simulink model "stm32f4_uart_hostpc_target_demo"  (Simulink 8.2)
settings: Solver=FixedStepDiscrete  SolverMode=SingleTasking  StartTime=0.0  StopTime=10.0  RelTol=1e-3
PreLoadFcn:
  | waijung.modelPreload; % Required for working with Waijung Blockset. Do not remove.
undefined symbols (not defined in the file): HSEOSC, Link, LQFP176, ST, STM32F417IG
libraries: stm32f4_io_lib x1, stm32f4_adc_lib x1, stm32f4_device_config_lib x1
CloseFcn:
  | waijung.modelClose; % Required for working with Waijung Blockset. Do not remove.
settings Model: Creator=Krisada  LastModifiedBy=Krisada
settings OptimizationCC: OptimizeModelRefInitCode=on  LifeSpan=1
settings DebuggingCC: ParameterPrecisionLossMsg=none
settings HardwareCC: ProdEndianess=LittleEndian  ProdHWDeviceType=ARM Compatible->Cortex - M4  TargetEndianess=LittleEndian  TargetHWDeviceType=ARM Compatible->Cortex - M4
settings RTWCC: SystemTargetFile=stm32f4.tlc  GenerateMakefile=off  TemplateMakefile=ert_default_tmf  Description=STM32F4 Target  ProcessScript=stm32f4_make_rtw_hook
settings CodeAppCC: IgnoreCustomStorageClasses=off  CustomSymbolStrType=$N$R$M  InternalIdentifier=Classic
settings STFCustomTargetCC: CodeReplacementLibrary=ANSI_C  ModelReferenceCompliant=off  CombineOutputUpdateFcns=on  ERTCustomFileBanners=on  SupportContinuousTime=off  SupportNonInlinedSFcns=off  MATLABClassNameForMDSCustomization=Simulink.SoftwareTarget.ERTCustomization  GRTInterface=off  SystemTargetFile=stm32f4.tlc
settings ERTTargetCC: CodeReplacementLibrary=ANSI_C  MultiwordLength=2048  ModelReferenceCompliant=off  ParMdlRefBuildCompliant=off  CompOptLevelCompliant=off  ConcurrentExecutionCompliant=off  ERTFirstTimeCompliant=off  ModelStepFunctionPrototypeControlCompliant=off  CPPClassGenCompliant=off  ExtModeMexFile=noextcomm  InlinedParameterPlacement=NonHierarchical  ERTSrcFileBannerTemplate=stm32f4_code_template.cgt  ERTHdrFileBannerTemplate=stm32f4_code_template.cgt  ERTDataSrcFileTemplate=stm32f4_code_template.cgt  ERTDataHdrFileTemplate=stm32f4_code_template.cgt  ERTCustomFileTemplate=stm32f4_file_process.tlc  ConvertIfToSwitch=off  SuppressUnreachableDefaultCases=off

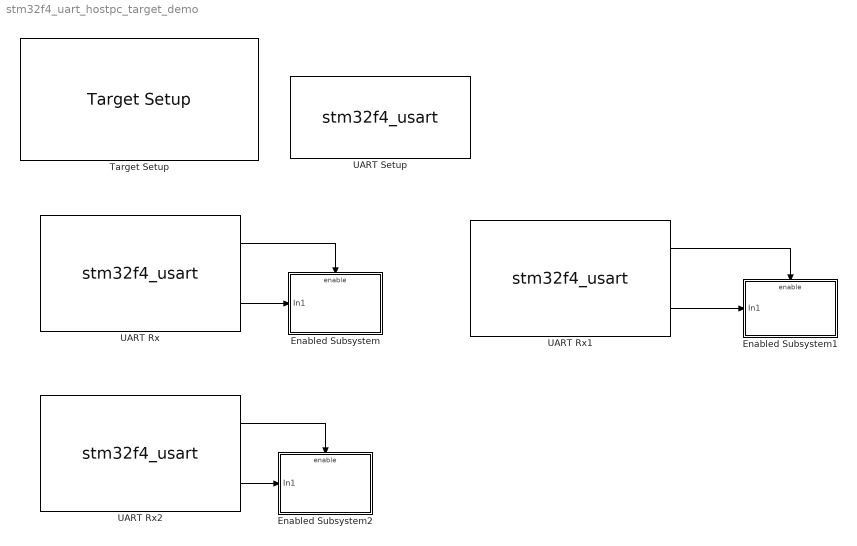
== system stm32f4_uart_hostpc_target_demo ==
  Enabled Subsystem : Subsystem  TreatAsAtomicUnit=on
  Enabled Subsystem1 : Subsystem  TreatAsAtomicUnit=on
  Enabled Subsystem2 : Subsystem  TreatAsAtomicUnit=on
  Target Setup : stm32f4_device_config_lib/Target Setup  Priority=100  compiler=GNU ARM  previous_compiler=GNU ARM  mcu=STM32F417IG (LQFP176)  mcustr=STM32F417IG  clockconfig=HSEOSC-8MHz  system_stm32f4xx_c_path=F:\trunk\targets\stm32f4_target\stm32f4\utils\system_stm32f4xx_default\STM32F40_41xxx\hseosc8mhz  showmemoryconfiguration=off  stacksize=0x400  heapsize=0x200  enableautocompiledownload=on  fullchiperase=off  programmerinterface=ST-Link  editctrlstr=on  compilercontrolstr=$(patsubst %, -I%, .) -mcpu=cortex-m4 -mthumb -mthumb-interwork -mfloat-abi=hard -mfpu=fpv4-sp-d16 -ffast-math -Wall -Wextra -Ofast  assemblercontrolstr=$(patsubst %, -I%, .) -mcpu=cortex-m4 -mthumb -mthumb-interwork -mfloat-abi=hard -mfpu=fpv4-sp-d16 -ffast-math -Wall -Wextra -Ofast -Wa,-amhls=$(<:.s=.lst) -D__STACK_SIZE=$(STACK_SIZE) -D__HEAP_SIZE=$(HEAP_SIZE)  linkercontrolstr=-T$(LD_SCRIPT) -g -Wl,-Map=$(MAP),--cref,--no-warn-mismatch -mcpu=cortex-m4 -mthumb -mthumb-interwork -mfloat-abi=hard -mfpu=fpv4-sp-d16 -specs=nosys.specs  runafterdownload=on  execprofile=None  profileruart=1  profilerbaud=115200  profilertxpin=D8  profilerinitstr=0.01,168000000,1680000,115200,0  manualsetsampletime=off  sampletime=0.01  blockid=TargetSetup  systickreloadvalue=1680000  hseval=8000000  lastprofileruart=1  hclk=168000000  flashorigin=0x8000000  flashlength=1024k  ramorigin=0x20000000  ramlength=128k  useextram=off
  UART Rx : S-Function  Priority=1  FunctionName=stm32f4_usart  Parameters=configuration,uartmodule,transfer,baudrate,inputtype,outputtype,confstr,binheaderarray,binterminatorarray,asciiheader,asciiterminator,bindatalength,packetmode,varname,sampletime,sampletimestr,blockid  EnableBusSupport=off  mask(stm32f4_usart){configuration=Rx, uartmodule=3, baudrate=115200, databits=8, parity=No, stopbit=1, remaptxpin=Not used, remaprxpin=Not used, flowcontrol=None, remapctspin=Not used, remaprtspin=Not used, advanceoptions=off, rxbuffersize=512, txbuffersize=512, transfer=Non-Blocking, packetmode=Ascii, binheader='7E 7E', binterminator='03 03', porttype_double=1, porttype_single=0, porttype_int8=1, porttype_uint8=0, porttype_int16=0, porttype_uint16=0, porttype_int32=0, porttype_uint32=0, asciiformat='LED1=%u', rx_asciiterminator=CR (0x0D - "\r"), tx_asciiterminator=LF (0x0A - "\n"), storagename=D0, varname=, inputtype=[0], outputtype=[2 3  7], binheaderarray=[0], binterminatorarray=[0], bindatalength=0, asciiheader='LED1=%u\r', asciiterminator=[1 13], sampletime=0.01, sampletimestr=0.01, blockid=UARTRx, confstr=[ "dummy", "0", "*", "*", "0", "*", "*", "0", "*", "*", "0", "*", "*", "1", "4", "3", "1", "4", "1", "512", "512", "1", "3", "115200", "8", "No", "1", "None", "USART3"], lastmodule=1}
      mask prompts: uartmodule "UART Module"; baudrate "Baud rate (bps)"; databits "Data bits"; stopbit "Stop bit"; remaptxpin "Tx Pin"; remaprxpin "Rx Pin"; flowcontrol "Hardware flow control"; remapctspin "HW Flow control, CTS Pin"; remaprtspin "HW Flow control, RTS Pin"; advanceoptions "Advance options"; rxbuffersize "Rx buffer size (bytes)"; txbuffersize "Tx buffer size (bytes)"; packetmode "Packet mode"; binheader "Binary header (example: '7E 7E')"; binterminator "Binary terminator (example: '03 03')"; porttype_double "Number of data port, type DOUBLE"; porttype_single "Number of data port, type SINGLE"; porttype_int8 "Number of data port, type INT8"; porttype_uint8 "Number of data port, type UINT8"; porttype_int16 "Number of data port, type INT16"; porttype_uint16 "Number of data port, type UINT16"; porttype_int32 "Number of data port, type INT32"; porttype_uint32 "Number of data port, type UINT32"; asciiformat "Ascii format"; rx_asciiterminator "End of packet"; tx_asciiterminator "End of packet"; storagename "Buffer"; varname "Var name"; inputtype "Input data type"; outputtype "Output data type"; binheaderarray "Binary header"; binterminatorarray "Binary terminator"; bindatalength "Binary data length"; asciiheader "Ascii header (printf format)"; asciiterminator "Ascii terminator"; sampletime "Sample time (sec)"; sampletimestr "Compiled sample time (sec) in string"; confstr "Configuration string"; lastmodule "Last module selected"
      mask init:
      | stm32f4_usart_callback('init');
      mask Help: web(fullfile(waijungdocroot,'stm32f4_usart_rx.htm'), '-browser')
      mask TypeOptions configuration: Setup | Tx | Rx
      mask Callback configuration: stm32f4_usart_callback('configuration');
      mask TypeOptions uartmodule: 1 | 2 | 3 | 4 | 5 | 6
      mask Callback uartmodule: stm32f4_usart_callback('uartmodule');
      mask Callback baudrate: stm32f4_usart_callback('baudrate');
      mask TypeOptions databits: 8
      mask TypeOptions parity: No | Odd | Even
      mask TypeOptions stopbit: 0.5 | 1 | 1.5 | 2
      mask TypeOptions remaptxpin: Not used | A9 | B6
      mask TypeOptions remaprxpin: Not used | A10 | B7
      mask TypeOptions flowcontrol: None | RTS | CTS | RTS/CTS
      mask Callback flowcontrol: stm32f4_usart_callback('flowcontrol');
      mask TypeOptions remapctspin: Not used | A11
      mask TypeOptions remaprtspin: Not used | A12
      mask Callback advanceoptions: stm32f4_usart_callback('advanceoptions');
      mask TypeOptions rxbuffersize: 16 | 32 | 64 | 128 | 256 | 512 | 1024 | 2048
      mask TypeOptions txbuffersize: 16 | 32 | 64 | 128 | 256 | 512 | 1024 | 2048
      mask TypeOptions transfer: Blocking | Non-Blocking
      mask Callback transfer: stm32f4_usart_callback('transfer');
      mask TypeOptions packetmode: Ascii | Binary | String Buffer
      mask Callback packetmode: stm32f4_usart_callback('packetmode');
      mask Callback binheader: stm32f4_usart_callback('binheader');
      mask Callback binterminator: stm32f4_usart_callback('binterminator');
      mask Callback porttype_double: stm32f4_usart_callback('porttype');
      mask Callback porttype_single: stm32f4_usart_callback('porttype');
      mask Callback porttype_int8: stm32f4_usart_callback('porttype');
      mask Callback porttype_uint8: stm32f4_usart_callback('porttype');
      mask Callback porttype_int16: stm32f4_usart_callback('porttype');
      mask Callback porttype_uint16: stm32f4_usart_callback('porttype');
      mask Callback porttype_int32: stm32f4_usart_callback('porttype');
      mask Callback porttype_uint32: stm32f4_usart_callback('porttype');
      mask Callback asciiformat: stm32f4_usart_callback('asciiformat');
      mask TypeOptions rx_asciiterminator: CR (0x0D - "\r") | LF (0x0A - "\n") | CRLF (0x0D 0x0A - "\r\n")
      mask Callback rx_asciiterminator: stm32f4_usart_callback('rx_asciiterminator');
      mask TypeOptions tx_asciiterminator: CR (0x0D - "\r") | LF (0x0A - "\n") | CRLF (0x0D 0x0A - "\r\n") | None
      mask Callback tx_asciiterminator: stm32f4_usart_callback('tx_asciiterminator');
      mask TypeOptions storagename: D0
      mask Callback storagename: stm32f4_usart_callback('storagename');
      mask Callback varname: stm32f4_usart_callback('varname');
      mask Callback sampletime: stm32f4_usart_callback('sampletime');
      mask Callback sampletimestr: stm32f4_usart_callback('sampletimestr');
      mask Callback blockid: stm32f4_usart_callback('blockid');
      mask Display: text(0.05, 0.5, 'Module: USART3_Rx\nPacket: Ascii\nTransfer: Non-Blocking\nTs (sec): 0.01','ver','middle','hor','left'); port_label('output', 1,'READY'); port_label('output', 2,'uint32');
  UART Rx1 : S-Function  Priority=1  FunctionName=stm32f4_usart  Parameters=configuration,uartmodule,transfer,baudrate,inputtype,outputtype,confstr,binheaderarray,binterminatorarray,asciiheader,asciiterminator,bindatalength,packetmode,varname,sampletime,sampletimestr,blockid  EnableBusSupport=off  mask(stm32f4_usart){configuration=Rx, uartmodule=3, baudrate=115200, databits=8, parity=No, stopbit=1, remaptxpin=Not used, remaprxpin=Not used, flowcontrol=None, remapctspin=Not used, remaprtspin=Not used, advanceoptions=off, rxbuffersize=512, txbuffersize=512, transfer=Non-Blocking, packetmode=Ascii, binheader='7E 7E', binterminator='03 03', porttype_double=1, porttype_single=0, porttype_int8=1, porttype_uint8=0, porttype_int16=0, porttype_uint16=0, porttype_int32=0, porttype_uint32=0, asciiformat='ADC%u?', rx_asciiterminator=CR (0x0D - "\r"), tx_asciiterminator=LF (0x0A - "\n"), storagename=<empty>, varname=, inputtype=[0], outputtype=[2 3  7], binheaderarray=[0], binterminatorarray=[0], bindatalength=0, asciiheader='ADC%u?\r', asciiterminator=[1 13], sampletime=0.01, sampletimestr=0.01, blockid=UARTRx1, confstr=[ "dummy", "0", "*", "*", "0", "*", "*", "0", "*", "*", "0", "*", "*", "1", "4", "3", "1", "4", "1", "512", "512", "1", "3", "115200", "8", "No", "1", "None", "USART3"], lastmodule=1}
      mask prompts: uartmodule "UART Module"; baudrate "Baud rate (bps)"; databits "Data bits"; stopbit "Stop bit"; remaptxpin "Tx Pin"; remaprxpin "Rx Pin"; flowcontrol "Hardware flow control"; remapctspin "HW Flow control, CTS Pin"; remaprtspin "HW Flow control, RTS Pin"; advanceoptions "Advance options"; rxbuffersize "Rx buffer size (bytes)"; txbuffersize "Tx buffer size (bytes)"; packetmode "Packet mode"; binheader "Binary header (example: '7E 7E')"; binterminator "Binary terminator (example: '03 03')"; porttype_double "Number of data port, type DOUBLE"; porttype_single "Number of data port, type SINGLE"; porttype_int8 "Number of data port, type INT8"; porttype_uint8 "Number of data port, type UINT8"; porttype_int16 "Number of data port, type INT16"; porttype_uint16 "Number of data port, type UINT16"; porttype_int32 "Number of data port, type INT32"; porttype_uint32 "Number of data port, type UINT32"; asciiformat "Ascii format"; rx_asciiterminator "End of packet"; tx_asciiterminator "End of packet"; storagename "Buffer"; varname "Var name"; inputtype "Input data type"; outputtype "Output data type"; binheaderarray "Binary header"; binterminatorarray "Binary terminator"; bindatalength "Binary data length"; asciiheader "Ascii header (printf format)"; asciiterminator "Ascii terminator"; sampletime "Sample time (sec)"; sampletimestr "Compiled sample time (sec) in string"; confstr "Configuration string"; lastmodule "Last module selected"
      mask init:
      | stm32f4_usart_callback('init');
      mask Help: web(fullfile(waijungdocroot,'stm32f4_usart_rx.htm'), '-browser')
      mask TypeOptions configuration: Setup | Tx | Rx
      mask Callback configuration: stm32f4_usart_callback('configuration');
      mask TypeOptions uartmodule: 1 | 2 | 3 | 4 | 5 | 6
      mask Callback uartmodule: stm32f4_usart_callback('uartmodule');
      mask Callback baudrate: stm32f4_usart_callback('baudrate');
      mask TypeOptions databits: 8
      mask TypeOptions parity: No | Odd | Even
      mask TypeOptions stopbit: 0.5 | 1 | 1.5 | 2
      mask TypeOptions remaptxpin: Not used | A9 | B6
      mask TypeOptions remaprxpin: Not used | A10 | B7
      mask TypeOptions flowcontrol: None | RTS | CTS | RTS/CTS
      mask Callback flowcontrol: stm32f4_usart_callback('flowcontrol');
      mask TypeOptions remapctspin: Not used | A11
      mask TypeOptions remaprtspin: Not used | A12
      mask Callback advanceoptions: stm32f4_usart_callback('advanceoptions');
      mask TypeOptions rxbuffersize: 16 | 32 | 64 | 128 | 256 | 512 | 1024 | 2048
      mask TypeOptions txbuffersize: 16 | 32 | 64 | 128 | 256 | 512 | 1024 | 2048
      mask TypeOptions transfer: Blocking | Non-Blocking
      mask Callback transfer: stm32f4_usart_callback('transfer');
      mask TypeOptions packetmode: Ascii | Binary | String Buffer
      mask Callback packetmode: stm32f4_usart_callback('packetmode');
      mask Callback binheader: stm32f4_usart_callback('binheader');
      mask Callback binterminator: stm32f4_usart_callback('binterminator');
      mask Callback porttype_double: stm32f4_usart_callback('porttype');
      mask Callback porttype_single: stm32f4_usart_callback('porttype');
      mask Callback porttype_int8: stm32f4_usart_callback('porttype');
      mask Callback porttype_uint8: stm32f4_usart_callback('porttype');
      mask Callback porttype_int16: stm32f4_usart_callback('porttype');
      mask Callback porttype_uint16: stm32f4_usart_callback('porttype');
      mask Callback porttype_int32: stm32f4_usart_callback('porttype');
      mask Callback porttype_uint32: stm32f4_usart_callback('porttype');
      mask Callback asciiformat: stm32f4_usart_callback('asciiformat');
      mask TypeOptions rx_asciiterminator: CR (0x0D - "\r") | LF (0x0A - "\n") | CRLF (0x0D 0x0A - "\r\n")
      mask Callback rx_asciiterminator: stm32f4_usart_callback('rx_asciiterminator');
      mask TypeOptions tx_asciiterminator: CR (0x0D - "\r") | LF (0x0A - "\n") | CRLF (0x0D 0x0A - "\r\n") | None
      mask Callback tx_asciiterminator: stm32f4_usart_callback('tx_asciiterminator');
      mask TypeOptions storagename: <empty>
      mask Callback storagename: stm32f4_usart_callback('storagename');
      mask Callback varname: stm32f4_usart_callback('varname');
      mask Callback sampletime: stm32f4_usart_callback('sampletime');
      mask Callback sampletimestr: stm32f4_usart_callback('sampletimestr');
      mask Callback blockid: stm32f4_usart_callback('blockid');
      mask Display: text(0.05, 0.5, 'Module: USART3_Rx\nPacket: Ascii\nTransfer: Non-Blocking\nTs (sec): 0.01','ver','middle','hor','left'); port_label('output', 1,'READY'); port_label('output', 2,'uint32');
  UART Rx2 : S-Function  Priority=1  FunctionName=stm32f4_usart  Parameters=configuration,uartmodule,transfer,baudrate,inputtype,outputtype,confstr,binheaderarray,binterminatorarray,asciiheader,asciiterminator,bindatalength,packetmode,varname,sampletime,sampletimestr,blockid  EnableBusSupport=off  mask(stm32f4_usart){configuration=Rx, uartmodule=3, baudrate=115200, databits=8, parity=No, stopbit=1, remaptxpin=Not used, remaprxpin=Not used, flowcontrol=None, remapctspin=Not used, remaprtspin=Not used, advanceoptions=off, rxbuffersize=512, txbuffersize=512, transfer=Non-Blocking, packetmode=Ascii, binheader='7E 7E', binterminator='03 03', porttype_double=1, porttype_single=0, porttype_int8=1, porttype_uint8=0, porttype_int16=0, porttype_uint16=0, porttype_int32=0, porttype_uint32=0, asciiformat='Input %f', rx_asciiterminator=CR (0x0D - "\r"), tx_asciiterminator=LF (0x0A - "\n"), storagename=<empty>, varname=, inputtype=[0], outputtype=[2 3  1], binheaderarray=[0], binterminatorarray=[0], bindatalength=0, asciiheader='Input %f\r', asciiterminator=[1 13], sampletime=0.01, sampletimestr=0.01, blockid=UARTRx2, confstr=[ "dummy", "0", "*", "*", "0", "*", "*", "0", "*", "*", "0", "*", "*", "1", "4", "3", "1", "4", "1", "512", "512", "1", "3", "115200", "8", "No", "1", "None", "USART3"], lastmodule=1}
      mask prompts: uartmodule "UART Module"; baudrate "Baud rate (bps)"; databits "Data bits"; stopbit "Stop bit"; remaptxpin "Tx Pin"; remaprxpin "Rx Pin"; flowcontrol "Hardware flow control"; remapctspin "HW Flow control, CTS Pin"; remaprtspin "HW Flow control, RTS Pin"; advanceoptions "Advance options"; rxbuffersize "Rx buffer size (bytes)"; txbuffersize "Tx buffer size (bytes)"; packetmode "Packet mode"; binheader "Binary header (example: '7E 7E')"; binterminator "Binary terminator (example: '03 03')"; porttype_double "Number of data port, type DOUBLE"; porttype_single "Number of data port, type SINGLE"; porttype_int8 "Number of data port, type INT8"; porttype_uint8 "Number of data port, type UINT8"; porttype_int16 "Number of data port, type INT16"; porttype_uint16 "Number of data port, type UINT16"; porttype_int32 "Number of data port, type INT32"; porttype_uint32 "Number of data port, type UINT32"; asciiformat "Ascii format"; rx_asciiterminator "End of packet"; tx_asciiterminator "End of packet"; storagename "Buffer"; varname "Var name"; inputtype "Input data type"; outputtype "Output data type"; binheaderarray "Binary header"; binterminatorarray "Binary terminator"; bindatalength "Binary data length"; asciiheader "Ascii header (printf format)"; asciiterminator "Ascii terminator"; sampletime "Sample time (sec)"; sampletimestr "Compiled sample time (sec) in string"; confstr "Configuration string"; lastmodule "Last module selected"
      mask init:
      | stm32f4_usart_callback('init');
      mask Help: web(fullfile(waijungdocroot,'stm32f4_usart_rx.htm'), '-browser')
      mask TypeOptions configuration: Setup | Tx | Rx
      mask Callback configuration: stm32f4_usart_callback('configuration');
      mask TypeOptions uartmodule: 1 | 2 | 3 | 4 | 5 | 6
      mask Callback uartmodule: stm32f4_usart_callback('uartmodule');
      mask Callback baudrate: stm32f4_usart_callback('baudrate');
      mask TypeOptions databits: 8
      mask TypeOptions parity: No | Odd | Even
      mask TypeOptions stopbit: 0.5 | 1 | 1.5 | 2
      mask TypeOptions remaptxpin: Not used | A9 | B6
      mask TypeOptions remaprxpin: Not used | A10 | B7
      mask TypeOptions flowcontrol: None | RTS | CTS | RTS/CTS
      mask Callback flowcontrol: stm32f4_usart_callback('flowcontrol');
      mask TypeOptions remapctspin: Not used | A11
      mask TypeOptions remaprtspin: Not used | A12
      mask Callback advanceoptions: stm32f4_usart_callback('advanceoptions');
      mask TypeOptions rxbuffersize: 16 | 32 | 64 | 128 | 256 | 512 | 1024 | 2048
      mask TypeOptions txbuffersize: 16 | 32 | 64 | 128 | 256 | 512 | 1024 | 2048
      mask TypeOptions transfer: Blocking | Non-Blocking
      mask Callback transfer: stm32f4_usart_callback('transfer');
      mask TypeOptions packetmode: Ascii | Binary | String Buffer
      mask Callback packetmode: stm32f4_usart_callback('packetmode');
      mask Callback binheader: stm32f4_usart_callback('binheader');
      mask Callback binterminator: stm32f4_usart_callback('binterminator');
      mask Callback porttype_double: stm32f4_usart_callback('porttype');
      mask Callback porttype_single: stm32f4_usart_callback('porttype');
      mask Callback porttype_int8: stm32f4_usart_callback('porttype');
      mask Callback porttype_uint8: stm32f4_usart_callback('porttype');
      mask Callback porttype_int16: stm32f4_usart_callback('porttype');
      mask Callback porttype_uint16: stm32f4_usart_callback('porttype');
      mask Callback porttype_int32: stm32f4_usart_callback('porttype');
      mask Callback porttype_uint32: stm32f4_usart_callback('porttype');
      mask Callback asciiformat: stm32f4_usart_callback('asciiformat');
      mask TypeOptions rx_asciiterminator: CR (0x0D - "\r") | LF (0x0A - "\n") | CRLF (0x0D 0x0A - "\r\n")
      mask Callback rx_asciiterminator: stm32f4_usart_callback('rx_asciiterminator');
      mask TypeOptions tx_asciiterminator: CR (0x0D - "\r") | LF (0x0A - "\n") | CRLF (0x0D 0x0A - "\r\n") | None
      mask Callback tx_asciiterminator: stm32f4_usart_callback('tx_asciiterminator');
      mask TypeOptions storagename: <empty>
      mask Callback storagename: stm32f4_usart_callback('storagename');
      mask Callback varname: stm32f4_usart_callback('varname');
      mask Callback sampletime: stm32f4_usart_callback('sampletime');
      mask Callback sampletimestr: stm32f4_usart_callback('sampletimestr');
      mask Callback blockid: stm32f4_usart_callback('blockid');
      mask Display: text(0.05, 0.5, 'Module: USART3_Rx\nPacket: Ascii\nTransfer: Non-Blocking\nTs (sec): 0.01','ver','middle','hor','left'); port_label('output', 1,'READY'); port_label('output', 2,'single');
  UART Setup : S-Function  Priority=1  FunctionName=stm32f4_usart  Parameters=configuration,uartmodule,transfer,baudrate,inputtype,outputtype,confstr,binheaderarray,binterminatorarray,asciiheader,asciiterminator,bindatalength,packetmode,varname,sampletime,sampletimestr,blockid  EnableBusSupport=off  mask(stm32f4_usart){configuration=Setup, uartmodule=3, baudrate=115200, databits=8, parity=No, stopbit=1, remaptxpin=D8, remaprxpin=D9, flowcontrol=None, remapctspin=Not used, remaprtspin=Not used, advanceoptions=off, rxbuffersize=512, txbuffersize=512, transfer=Blocking, packetmode=Ascii, binheader='7E 7E', binterminator='03 03', porttype_double=1, porttype_single=0, porttype_int8=1, porttype_uint8=0, porttype_int16=0, porttype_uint16=0, porttype_int32=0, porttype_uint32=0, asciiformat='%d,%f', rx_asciiterminator=CRLF (0x0D 0x0A - "\r\n"), tx_asciiterminator=CR (0x0D - "\r"), storagename=<empty>, varname=, inputtype=[0], outputtype=[0], binheaderarray=[0], binterminatorarray=[0], bindatalength=0, asciiheader='', asciiterminator=[0], sampletime=-1, sampletimestr=0.01, blockid=UARTSetup, confstr=[ "dummy", "1", "D", "8", "1", "D", "9", "0", "*", "*", "0", "*", "*", "1", "4", "3", "1", "4", "1", "512", "512", "1", "3", "115200", "8", "No", "1", "None", "USART3"], lastmodule=3}
      mask prompts: uartmodule "UART Module"; baudrate "Baud rate (bps)"; databits "Data bits"; stopbit "Stop bit"; remaptxpin "Tx Pin"; remaprxpin "Rx Pin"; flowcontrol "Hardware flow control"; remapctspin "HW Flow control, CTS Pin"; remaprtspin "HW Flow control, RTS Pin"; advanceoptions "Advance options"; rxbuffersize "Rx buffer size (bytes)"; txbuffersize "Tx buffer size (bytes)"; packetmode "Packet mode"; binheader "Binary header (example: '7E 7E')"; binterminator "Binary terminator (example: '03 03')"; porttype_double "Number of data port, type DOUBLE"; porttype_single "Number of data port, type SINGLE"; porttype_int8 "Number of data port, type INT8"; porttype_uint8 "Number of data port, type UINT8"; porttype_int16 "Number of data port, type INT16"; porttype_uint16 "Number of data port, type UINT16"; porttype_int32 "Number of data port, type INT32"; porttype_uint32 "Number of data port, type UINT32"; asciiformat "Ascii format"; rx_asciiterminator "End of packet"; tx_asciiterminator "End of packet"; storagename "Buffer"; varname "Var name"; inputtype "Input data type"; outputtype "Output data type"; binheaderarray "Binary header"; binterminatorarray "Binary terminator"; bindatalength "Binary data length"; asciiheader "Ascii header (printf format)"; asciiterminator "Ascii terminator"; sampletime "Sample time (sec)"; sampletimestr "Compiled sample time (sec) in string"; confstr "Configuration string"; lastmodule "Last module selected"
      mask init:
      | stm32f4_usart_callback('init');
      mask Help: web(fullfile(waijungdocroot,'stm32f4_usart_setup.htm'), '-browser')
      mask TypeOptions configuration: Setup | Tx | Rx
      mask Callback configuration: stm32f4_usart_callback('configuration');
      mask TypeOptions uartmodule: 1 | 2 | 3 | 4 | 5 | 6
      mask Callback uartmodule: stm32f4_usart_callback('uartmodule');
      mask Callback baudrate: stm32f4_usart_callback('baudrate');
      mask TypeOptions databits: 8
      mask TypeOptions parity: No | Odd | Even
      mask TypeOptions stopbit: 0.5 | 1 | 1.5 | 2
      mask TypeOptions remaptxpin: Not used | B10 | C10 | D8
      mask TypeOptions remaprxpin: Not used | B11 | C11 | D9
      mask TypeOptions flowcontrol: None | RTS | CTS | RTS/CTS
      mask Callback flowcontrol: stm32f4_usart_callback('flowcontrol');
      mask TypeOptions remapctspin: Not used | B13 | D11
      mask TypeOptions remaprtspin: Not used | B14 | D12
      mask Callback advanceoptions: stm32f4_usart_callback('advanceoptions');
      mask TypeOptions rxbuffersize: 16 | 32 | 64 | 128 | 256 | 512 | 1024 | 2048
      mask TypeOptions txbuffersize: 16 | 32 | 64 | 128 | 256 | 512 | 1024 | 2048
      mask TypeOptions transfer: Blocking | Non-Blocking
      mask Callback transfer: stm32f4_usart_callback('transfer');
      mask TypeOptions packetmode: Ascii | Binary | String Buffer
      mask Callback packetmode: stm32f4_usart_callback('packetmode');
      mask Callback binheader: stm32f4_usart_callback('binheader');
      mask Callback binterminator: stm32f4_usart_callback('binterminator');
      mask Callback porttype_double: stm32f4_usart_callback('porttype');
      mask Callback porttype_single: stm32f4_usart_callback('porttype');
      mask Callback porttype_int8: stm32f4_usart_callback('porttype');
      mask Callback porttype_uint8: stm32f4_usart_callback('porttype');
      mask Callback porttype_int16: stm32f4_usart_callback('porttype');
      mask Callback porttype_uint16: stm32f4_usart_callback('porttype');
      mask Callback porttype_int32: stm32f4_usart_callback('porttype');
      mask Callback porttype_uint32: stm32f4_usart_callback('porttype');
      mask Callback asciiformat: stm32f4_usart_callback('asciiformat');
      mask TypeOptions rx_asciiterminator: CR (0x0D - "\r") | LF (0x0A - "\n") | CRLF (0x0D 0x0A - "\r\n")
      mask Callback rx_asciiterminator: stm32f4_usart_callback('rx_asciiterminator');
      mask TypeOptions tx_asciiterminator: CR (0x0D - "\r") | LF (0x0A - "\n") | CRLF (0x0D 0x0A - "\r\n") | None
      mask Callback tx_asciiterminator: stm32f4_usart_callback('tx_asciiterminator');
      mask TypeOptions storagename: <empty>
      mask Callback storagename: stm32f4_usart_callback('storagename');
      mask Callback varname: stm32f4_usart_callback('varname');
      mask Callback sampletime: stm32f4_usart_callback('sampletime');
      mask Callback sampletimestr: stm32f4_usart_callback('sampletimestr');
      mask Callback blockid: stm32f4_usart_callback('blockid');
      mask Display: text(0.5, 0.5, 'Module: USART3_Setup\nBaud (Bps): 115200\nDMA Buffer: 512/512\nTx/Rx Pin: D8/D9','ver','middle','hor','center');
  wires:
  UART Rx1/1 -> Enabled Subsystem1/Enable
  UART Rx1/2 -> Enabled Subsystem1/1(In1)
  UART Rx2/2 -> Enabled Subsystem2/1(In1)
  UART Rx2/1 -> Enabled Subsystem2/Enable
  UART Rx/1 -> Enabled Subsystem/Enable
  UART Rx/2 -> Enabled Subsystem/1(In1)

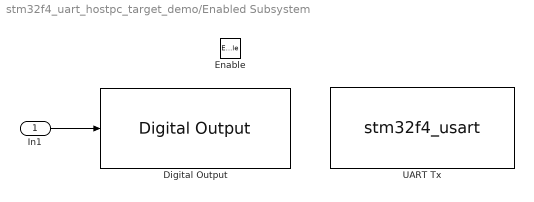
== system stm32f4_uart_hostpc_target_demo/Enabled Subsystem ==
  In1 : Inport
  Enable : EnablePort  PropagateVarSize=During execution
  Digital Output : stm32f4_io_lib/Digital Output  use_bitband=on  port=D  speed=100  porttype=Push Pull  porttypestr=PP  use_pin0=off  use_pin1=off  use_pin2=off  use_pin3=off  use_pin4=off  use_pin5=off  use_pin6=off  use_pin7=off  use_pin8=off  use_pin9=off  use_pin10=off  use_pin11=off  use_pin12=on  use_pin13=off  use_pin14=off  use_pin15=off  pinstr=GPIO_Pin_12  usedpinarray="[0  0  0  0  0  0  0  0  0  0  0  0  1  0  0  0]"  bitbandingstr="#define EnabledSubsystemDigitalOutput_D12 Peripheral_BB(GPIOD->ODR, 12)  /* Output pin */"  sampletime=-1  sampletimestr=0.01  blockid=EnabledSubsystemDigitalOutput  enablecustomportlabel=off  globalinit=off  cinputportlabel=In1, In2  coutputportlabel=0
  UART Tx : S-Function  Priority=1  FunctionName=stm32f4_usart  Parameters=configuration,uartmodule,transfer,baudrate,inputtype,outputtype,confstr,binheaderarray,binterminatorarray,asciiheader,asciiterminator,bindatalength,packetmode,varname,sampletime,sampletimestr,blockid  EnableBusSupport=off  mask(stm32f4_usart){configuration=Tx, uartmodule=3, baudrate=115200, databits=8, parity=No, stopbit=1, remaptxpin=Not used, remaprxpin=Not used, flowcontrol=None, remapctspin=Not used, remaprtspin=Not used, advanceoptions=off, rxbuffersize=512, txbuffersize=512, transfer=Blocking, packetmode=Ascii, binheader='7E 7E', binterminator='03 03', porttype_double=1, porttype_single=0, porttype_int8=1, porttype_uint8=0, porttype_int16=0, porttype_uint16=0, porttype_int32=0, porttype_uint32=0, asciiformat='Ok', rx_asciiterminator=CRLF (0x0D 0x0A - "\r\n"), tx_asciiterminator=CRLF (0x0D 0x0A - "\r\n"), storagename=<empty>, varname=, inputtype=[0 ], outputtype=[0], binheaderarray=[0], binterminatorarray=[0], bindatalength=0, asciiheader='Ok\r\n', asciiterminator=[2 13 10], sampletime=-1, sampletimestr=0.01, blockid=EnabledSubsystemUARTTx, confstr=[ "dummy", "0", "*", "*", "0", "*", "*", "0", "*", "*", "0", "*", "*", "1", "4", "3", "1", "4", "1", "512", "512", "1", "3", "115200", "8", "No", "1", "None", "USART3"], lastmodule=1}
      mask prompts: uartmodule "UART Module"; baudrate "Baud rate (bps)"; databits "Data bits"; stopbit "Stop bit"; remaptxpin "Tx Pin"; remaprxpin "Rx Pin"; flowcontrol "Hardware flow control"; remapctspin "HW Flow control, CTS Pin"; remaprtspin "HW Flow control, RTS Pin"; advanceoptions "Advance options"; rxbuffersize "Rx buffer size (bytes)"; txbuffersize "Tx buffer size (bytes)"; packetmode "Packet mode"; binheader "Binary header (example: '7E 7E')"; binterminator "Binary terminator (example: '03 03')"; porttype_double "Number of data port, type DOUBLE"; porttype_single "Number of data port, type SINGLE"; porttype_int8 "Number of data port, type INT8"; porttype_uint8 "Number of data port, type UINT8"; porttype_int16 "Number of data port, type INT16"; porttype_uint16 "Number of data port, type UINT16"; porttype_int32 "Number of data port, type INT32"; porttype_uint32 "Number of data port, type UINT32"; asciiformat "Ascii format"; rx_asciiterminator "End of packet"; tx_asciiterminator "End of packet"; storagename "Buffer"; varname "Var name"; inputtype "Input data type"; outputtype "Output data type"; binheaderarray "Binary header"; binterminatorarray "Binary terminator"; bindatalength "Binary data length"; asciiheader "Ascii header (printf format)"; asciiterminator "Ascii terminator"; sampletime "Sample time (sec)"; sampletimestr "Compiled sample time (sec) in string"; confstr "Configuration string"; lastmodule "Last module selected"
      mask init:
      | stm32f4_usart_callback('init');
      mask Help: web(fullfile(waijungdocroot,'stm32f4_usart_tx.htm'), '-browser')
      mask TypeOptions configuration: Setup | Tx | Rx
      mask Callback configuration: stm32f4_usart_callback('configuration');
      mask TypeOptions uartmodule: 1 | 2 | 3 | 4 | 5 | 6
      mask Callback uartmodule: stm32f4_usart_callback('uartmodule');
      mask Callback baudrate: stm32f4_usart_callback('baudrate');
      mask TypeOptions databits: 8
      mask TypeOptions parity: No | Odd | Even
      mask TypeOptions stopbit: 0.5 | 1 | 1.5 | 2
      mask TypeOptions remaptxpin: Not used | A9 | B6
      mask TypeOptions remaprxpin: Not used | A10 | B7
      mask TypeOptions flowcontrol: None | RTS | CTS | RTS/CTS
      mask Callback flowcontrol: stm32f4_usart_callback('flowcontrol');
      mask TypeOptions remapctspin: Not used | A11
      mask TypeOptions remaprtspin: Not used | A12
      mask Callback advanceoptions: stm32f4_usart_callback('advanceoptions');
      mask TypeOptions rxbuffersize: 16 | 32 | 64 | 128 | 256 | 512 | 1024 | 2048
      mask TypeOptions txbuffersize: 16 | 32 | 64 | 128 | 256 | 512 | 1024 | 2048
      mask TypeOptions transfer: Blocking | Non-Blocking
      mask Callback transfer: stm32f4_usart_callback('transfer');
      mask TypeOptions packetmode: Ascii | Binary | String Buffer
      mask Callback packetmode: stm32f4_usart_callback('packetmode');
      mask Callback binheader: stm32f4_usart_callback('binheader');
      mask Callback binterminator: stm32f4_usart_callback('binterminator');
      mask Callback porttype_double: stm32f4_usart_callback('porttype');
      mask Callback porttype_single: stm32f4_usart_callback('porttype');
      mask Callback porttype_int8: stm32f4_usart_callback('porttype');
      mask Callback porttype_uint8: stm32f4_usart_callback('porttype');
      mask Callback porttype_int16: stm32f4_usart_callback('porttype');
      mask Callback porttype_uint16: stm32f4_usart_callback('porttype');
      mask Callback porttype_int32: stm32f4_usart_callback('porttype');
      mask Callback porttype_uint32: stm32f4_usart_callback('porttype');
      mask Callback asciiformat: stm32f4_usart_callback('asciiformat');
      mask TypeOptions rx_asciiterminator: CR (0x0D - "\r") | LF (0x0A - "\n") | CRLF (0x0D 0x0A - "\r\n")
      mask Callback rx_asciiterminator: stm32f4_usart_callback('rx_asciiterminator');
      mask TypeOptions tx_asciiterminator: CR (0x0D - "\r") | LF (0x0A - "\n") | CRLF (0x0D 0x0A - "\r\n") | None
      mask Callback tx_asciiterminator: stm32f4_usart_callback('tx_asciiterminator');
      mask TypeOptions storagename: <empty>
      mask Callback storagename: stm32f4_usart_callback('storagename');
      mask Callback varname: stm32f4_usart_callback('varname');
      mask Callback sampletime: stm32f4_usart_callback('sampletime');
      mask Callback sampletimestr: stm32f4_usart_callback('sampletimestr');
      mask Callback blockid: stm32f4_usart_callback('blockid');
      mask Display: text(0.95, 0.5, 'Module: USART3_Tx\nPacket: Ascii\nTransfer: Blocking\nTs (sec): 0.01','ver','middle','hor','right');
  wires:
  In1/1 -> Digital Output/1

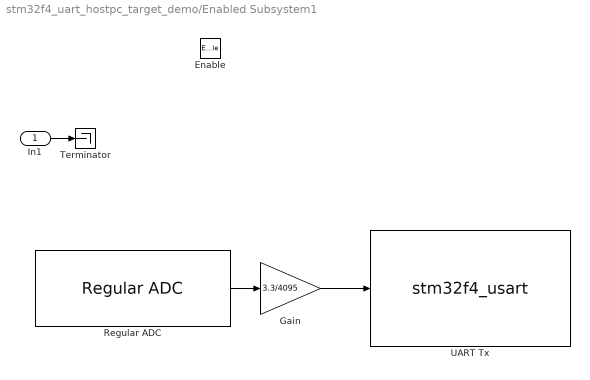
== system stm32f4_uart_hostpc_target_demo/Enabled Subsystem1 ==
  In1 : Inport
  Enable : EnablePort  PropagateVarSize=During execution
  Gain : Gain  Gain=3.3/4095  ParamDataTypeStr=single  OutDataTypeStr=single
  Regular ADC : stm32f4_adc_lib/Regular ADC  adcmodule=1  outputdatatype=Single  prescaler=2  prescalerstr=ADC_Prescaler_Div2  chsamplingtime=Auto  chsamplingtimestr=ADC_SampleTime_480Cycles  read_an0=on  read_an1=off  read_an2=off  read_an3=off  read_an4=off  read_an5=off  read_an6=off  read_an7=off  read_an8=off  read_an9=off  read_an10=off  read_an11=off  read_an12=off  read_an13=off  read_an14=off  read_an15=off  read_an16=off  read_an17=off  read_an18=off  pinstr=GPIO_Pin_0  usedpinarray="[1  0  0  0  0  0  0  0  0  0  0  0  0  0  0  0  0  0  0]"  usedportidarray=[0]  usedpinidarray=[0]  usedpinidcount=1  sampletime=0.01  blockid=EnabledSubsystem1RegularADC  enablecustomportlabel=off  cinputportlabel=0  coutputportlabel=Out1, Out2
  Terminator : Terminator
  UART Tx : S-Function  Priority=1  FunctionName=stm32f4_usart  Parameters=configuration,uartmodule,transfer,baudrate,inputtype,outputtype,confstr,binheaderarray,binterminatorarray,asciiheader,asciiterminator,bindatalength,packetmode,varname,sampletime,sampletimestr,blockid  EnableBusSupport=off  mask(stm32f4_usart){configuration=Tx, uartmodule=3, baudrate=115200, databits=8, parity=No, stopbit=1, remaptxpin=Not used, remaprxpin=Not used, flowcontrol=None, remapctspin=Not used, remaprtspin=Not used, advanceoptions=off, rxbuffersize=512, txbuffersize=512, transfer=Blocking, packetmode=Ascii, binheader='7E 7E', binterminator='03 03', porttype_double=1, porttype_single=0, porttype_int8=1, porttype_uint8=0, porttype_int16=0, porttype_uint16=0, porttype_int32=0, porttype_uint32=0, asciiformat='Reading=%f', rx_asciiterminator=CRLF (0x0D 0x0A - "\r\n"), tx_asciiterminator=CRLF (0x0D 0x0A - "\r\n"), storagename=<empty>, varname=, inputtype=[1  1], outputtype=[0], binheaderarray=[0], binterminatorarray=[0], bindatalength=0, asciiheader='Reading=%f\r\n', asciiterminator=[2 13 10], sampletime=-1, sampletimestr=0.01, blockid=EnabledSubsystem1UARTTx, confstr=[ "dummy", "0", "*", "*", "0", "*", "*", "0", "*", "*", "0", "*", "*", "1", "4", "3", "1", "4", "1", "512", "512", "1", "3", "115200", "8", "No", "1", "None", "USART3"], lastmodule=1}
      mask prompts: uartmodule "UART Module"; baudrate "Baud rate (bps)"; databits "Data bits"; stopbit "Stop bit"; remaptxpin "Tx Pin"; remaprxpin "Rx Pin"; flowcontrol "Hardware flow control"; remapctspin "HW Flow control, CTS Pin"; remaprtspin "HW Flow control, RTS Pin"; advanceoptions "Advance options"; rxbuffersize "Rx buffer size (bytes)"; txbuffersize "Tx buffer size (bytes)"; packetmode "Packet mode"; binheader "Binary header (example: '7E 7E')"; binterminator "Binary terminator (example: '03 03')"; porttype_double "Number of data port, type DOUBLE"; porttype_single "Number of data port, type SINGLE"; porttype_int8 "Number of data port, type INT8"; porttype_uint8 "Number of data port, type UINT8"; porttype_int16 "Number of data port, type INT16"; porttype_uint16 "Number of data port, type UINT16"; porttype_int32 "Number of data port, type INT32"; porttype_uint32 "Number of data port, type UINT32"; asciiformat "Ascii format"; rx_asciiterminator "End of packet"; tx_asciiterminator "End of packet"; storagename "Buffer"; varname "Var name"; inputtype "Input data type"; outputtype "Output data type"; binheaderarray "Binary header"; binterminatorarray "Binary terminator"; bindatalength "Binary data length"; asciiheader "Ascii header (printf format)"; asciiterminator "Ascii terminator"; sampletime "Sample time (sec)"; sampletimestr "Compiled sample time (sec) in string"; confstr "Configuration string"; lastmodule "Last module selected"
      mask init:
      | stm32f4_usart_callback('init');
      mask Help: web(fullfile(waijungdocroot,'stm32f4_usart_tx.htm'), '-browser')
      mask TypeOptions configuration: Setup | Tx | Rx
      mask Callback configuration: stm32f4_usart_callback('configuration');
      mask TypeOptions uartmodule: 1 | 2 | 3 | 4 | 5 | 6
      mask Callback uartmodule: stm32f4_usart_callback('uartmodule');
      mask Callback baudrate: stm32f4_usart_callback('baudrate');
      mask TypeOptions databits: 8
      mask TypeOptions parity: No | Odd | Even
      mask TypeOptions stopbit: 0.5 | 1 | 1.5 | 2
      mask TypeOptions remaptxpin: Not used | A9 | B6
      mask TypeOptions remaprxpin: Not used | A10 | B7
      mask TypeOptions flowcontrol: None | RTS | CTS | RTS/CTS
      mask Callback flowcontrol: stm32f4_usart_callback('flowcontrol');
      mask TypeOptions remapctspin: Not used | A11
      mask TypeOptions remaprtspin: Not used | A12
      mask Callback advanceoptions: stm32f4_usart_callback('advanceoptions');
      mask TypeOptions rxbuffersize: 16 | 32 | 64 | 128 | 256 | 512 | 1024 | 2048
      mask TypeOptions txbuffersize: 16 | 32 | 64 | 128 | 256 | 512 | 1024 | 2048
      mask TypeOptions transfer: Blocking | Non-Blocking
      mask Callback transfer: stm32f4_usart_callback('transfer');
      mask TypeOptions packetmode: Ascii | Binary | String Buffer
      mask Callback packetmode: stm32f4_usart_callback('packetmode');
      mask Callback binheader: stm32f4_usart_callback('binheader');
      mask Callback binterminator: stm32f4_usart_callback('binterminator');
      mask Callback porttype_double: stm32f4_usart_callback('porttype');
      mask Callback porttype_single: stm32f4_usart_callback('porttype');
      mask Callback porttype_int8: stm32f4_usart_callback('porttype');
      mask Callback porttype_uint8: stm32f4_usart_callback('porttype');
      mask Callback porttype_int16: stm32f4_usart_callback('porttype');
      mask Callback porttype_uint16: stm32f4_usart_callback('porttype');
      mask Callback porttype_int32: stm32f4_usart_callback('porttype');
      mask Callback porttype_uint32: stm32f4_usart_callback('porttype');
      mask Callback asciiformat: stm32f4_usart_callback('asciiformat');
      mask TypeOptions rx_asciiterminator: CR (0x0D - "\r") | LF (0x0A - "\n") | CRLF (0x0D 0x0A - "\r\n")
      mask Callback rx_asciiterminator: stm32f4_usart_callback('rx_asciiterminator');
      mask TypeOptions tx_asciiterminator: CR (0x0D - "\r") | LF (0x0A - "\n") | CRLF (0x0D 0x0A - "\r\n") | None
      mask Callback tx_asciiterminator: stm32f4_usart_callback('tx_asciiterminator');
      mask TypeOptions storagename: <empty>
      mask Callback storagename: stm32f4_usart_callback('storagename');
      mask Callback varname: stm32f4_usart_callback('varname');
      mask Callback sampletime: stm32f4_usart_callback('sampletime');
      mask Callback sampletimestr: stm32f4_usart_callback('sampletimestr');
      mask Callback blockid: stm32f4_usart_callback('blockid');
      mask Display: text(0.95, 0.5, 'Module: USART3_Tx\nPacket: Ascii\nTransfer: Blocking\nTs (sec): 0.01','ver','middle','hor','right'); port_label('input', 1,'single');
  wires:
  In1/1 -> Terminator/1
  Gain/1 -> UART Tx/1
  Regular ADC/1 -> Gain/1

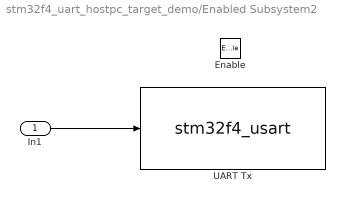
== system stm32f4_uart_hostpc_target_demo/Enabled Subsystem2 ==
  In1 : Inport
  Enable : EnablePort  PropagateVarSize=During execution
  UART Tx : S-Function  Priority=1  FunctionName=stm32f4_usart  Parameters=configuration,uartmodule,transfer,baudrate,inputtype,outputtype,confstr,binheaderarray,binterminatorarray,asciiheader,asciiterminator,bindatalength,packetmode,varname,sampletime,sampletimestr,blockid  EnableBusSupport=off  mask(stm32f4_usart){configuration=Tx, uartmodule=3, baudrate=115200, databits=8, parity=No, stopbit=1, remaptxpin=Not used, remaprxpin=Not used, flowcontrol=None, remapctspin=Not used, remaprtspin=Not used, advanceoptions=off, rxbuffersize=512, txbuffersize=512, transfer=Blocking, packetmode=Ascii, binheader='7E 7E', binterminator='03 03', porttype_double=1, porttype_single=0, porttype_int8=1, porttype_uint8=0, porttype_int16=0, porttype_uint16=0, porttype_int32=0, porttype_uint32=0, asciiformat='>>Your input is: %f', rx_asciiterminator=CRLF (0x0D 0x0A - "\r\n"), tx_asciiterminator=CRLF (0x0D 0x0A - "\r\n"), storagename=<empty>, varname=, inputtype=[1  1], outputtype=[0], binheaderarray=[0], binterminatorarray=[0], bindatalength=0, asciiheader='>>Your input is: %f\r\n', asciiterminator=[2 13 10], sampletime=-1, sampletimestr=0.01, blockid=EnabledSubsystem2UARTTx, confstr=[ "dummy", "0", "*", "*", "0", "*", "*", "0", "*", "*", "0", "*", "*", "1", "4", "3", "1", "4", "1", "512", "512", "1", "3", "115200", "8", "No", "1", "None", "USART3"], lastmodule=1}
      mask prompts: uartmodule "UART Module"; baudrate "Baud rate (bps)"; databits "Data bits"; stopbit "Stop bit"; remaptxpin "Tx Pin"; remaprxpin "Rx Pin"; flowcontrol "Hardware flow control"; remapctspin "HW Flow control, CTS Pin"; remaprtspin "HW Flow control, RTS Pin"; advanceoptions "Advance options"; rxbuffersize "Rx buffer size (bytes)"; txbuffersize "Tx buffer size (bytes)"; packetmode "Packet mode"; binheader "Binary header (example: '7E 7E')"; binterminator "Binary terminator (example: '03 03')"; porttype_double "Number of data port, type DOUBLE"; porttype_single "Number of data port, type SINGLE"; porttype_int8 "Number of data port, type INT8"; porttype_uint8 "Number of data port, type UINT8"; porttype_int16 "Number of data port, type INT16"; porttype_uint16 "Number of data port, type UINT16"; porttype_int32 "Number of data port, type INT32"; porttype_uint32 "Number of data port, type UINT32"; asciiformat "Ascii format"; rx_asciiterminator "End of packet"; tx_asciiterminator "End of packet"; storagename "Buffer"; varname "Var name"; inputtype "Input data type"; outputtype "Output data type"; binheaderarray "Binary header"; binterminatorarray "Binary terminator"; bindatalength "Binary data length"; asciiheader "Ascii header (printf format)"; asciiterminator "Ascii terminator"; sampletime "Sample time (sec)"; sampletimestr "Compiled sample time (sec) in string"; confstr "Configuration string"; lastmodule "Last module selected"
      mask init:
      | stm32f4_usart_callback('init');
      mask Help: web(fullfile(waijungdocroot,'stm32f4_usart_tx.htm'), '-browser')
      mask TypeOptions configuration: Setup | Tx | Rx
      mask Callback configuration: stm32f4_usart_callback('configuration');
      mask TypeOptions uartmodule: 1 | 2 | 3 | 4 | 5 | 6
      mask Callback uartmodule: stm32f4_usart_callback('uartmodule');
      mask Callback baudrate: stm32f4_usart_callback('baudrate');
      mask TypeOptions databits: 8
      mask TypeOptions parity: No | Odd | Even
      mask TypeOptions stopbit: 0.5 | 1 | 1.5 | 2
      mask TypeOptions remaptxpin: Not used | A9 | B6
      mask TypeOptions remaprxpin: Not used | A10 | B7
      mask TypeOptions flowcontrol: None | RTS | CTS | RTS/CTS
      mask Callback flowcontrol: stm32f4_usart_callback('flowcontrol');
      mask TypeOptions remapctspin: Not used | A11
      mask TypeOptions remaprtspin: Not used | A12
      mask Callback advanceoptions: stm32f4_usart_callback('advanceoptions');
      mask TypeOptions rxbuffersize: 16 | 32 | 64 | 128 | 256 | 512 | 1024 | 2048
      mask TypeOptions txbuffersize: 16 | 32 | 64 | 128 | 256 | 512 | 1024 | 2048
      mask TypeOptions transfer: Blocking | Non-Blocking
      mask Callback transfer: stm32f4_usart_callback('transfer');
      mask TypeOptions packetmode: Ascii | Binary | String Buffer
      mask Callback packetmode: stm32f4_usart_callback('packetmode');
      mask Callback binheader: stm32f4_usart_callback('binheader');
      mask Callback binterminator: stm32f4_usart_callback('binterminator');
      mask Callback porttype_double: stm32f4_usart_callback('porttype');
      mask Callback porttype_single: stm32f4_usart_callback('porttype');
      mask Callback porttype_int8: stm32f4_usart_callback('porttype');
      mask Callback porttype_uint8: stm32f4_usart_callback('porttype');
      mask Callback porttype_int16: stm32f4_usart_callback('porttype');
      mask Callback porttype_uint16: stm32f4_usart_callback('porttype');
      mask Callback porttype_int32: stm32f4_usart_callback('porttype');
      mask Callback porttype_uint32: stm32f4_usart_callback('porttype');
      mask Callback asciiformat: stm32f4_usart_callback('asciiformat');
      mask TypeOptions rx_asciiterminator: CR (0x0D - "\r") | LF (0x0A - "\n") | CRLF (0x0D 0x0A - "\r\n")
      mask Callback rx_asciiterminator: stm32f4_usart_callback('rx_asciiterminator');
      mask TypeOptions tx_asciiterminator: CR (0x0D - "\r") | LF (0x0A - "\n") | CRLF (0x0D 0x0A - "\r\n") | None
      mask Callback tx_asciiterminator: stm32f4_usart_callback('tx_asciiterminator');
      mask TypeOptions storagename: <empty>
      mask Callback storagename: stm32f4_usart_callback('storagename');
      mask Callback varname: stm32f4_usart_callback('varname');
      mask Callback sampletime: stm32f4_usart_callback('sampletime');
      mask Callback sampletimestr: stm32f4_usart_callback('sampletimestr');
      mask Callback blockid: stm32f4_usart_callback('blockid');
      mask Display: text(0.95, 0.5, 'Module: USART3_Tx\nPacket: Ascii\nTransfer: Blocking\nTs (sec): 0.01','ver','middle','hor','right'); port_label('input', 1,'single');
  wires:
  In1/1 -> UART Tx/1
